simulink library "Arithmetic_Operations_Lib"  (R2023a)
settings: Solver=ode45  StartTime=0.0  StopTime=10.0  RelTol=1e-3  EnableMultiTasking=on
libraries: Miscellaneous x202
(part 1 of 4)
settings Model: Creator=uzivatel  LastModifiedBy=Jozko Mrkvicka
settings SolverCC: AlgebraicLoopSolver=TrustRegion
settings DataIOCC: LimitDataPoints=on  SaveFormat=Array  ReturnWorkspaceOutputs=off
settings OptimizationCC: LifeSpan=inf
settings DebuggingCC: UnderspecifiedInitializationDetection=Classic  MergeDetectMultiDrivingBlocksExec=none  SolverPrmCheckMsg=warning  UnconnectedInputMsg=warning  UnconnectedOutputMsg=warning  UnconnectedLineMsg=warning  StateNameClashWarn=warning  SFUnexpectedBacktrackingDiag=warning  SFNoUnconditionalDefaultTransitionDiag=warning  ArithmeticOperatorsInVariantConditions=warning
settings HardwareCC: ProdBitPerPointer=32  ProdBitPerSizeT=32  ProdBitPerPtrDiffT=32  ProdLargestAtomicFloat=None  ProdIntDivRoundTo=Undefined  ProdEndianess=Unspecified  ProdWordSize=32  ProdHWDeviceType=32-bit Generic
settings ModelReferenceCC: EnableRefExpFcnMdlSchedulingChecks=on  PropagateSignalLabelsOutOfModel=off
settings SFSimCC: SimUseLocalCustomCode=off  CustomCodeUndefinedFunction=UseInterfaceOnly
settings RTWCC: RTWUseLocalCustomCode=off
settings CodeAppCC: StateflowObjectComments=on
settings GRTTargetCC: TargetLangStandard=C89/C90 (ANSI)
settings ConfigComp: CovMetricSettings=dw  CovSaveCumulativeToWorkspaceVar=on  CovSaveSingleToWorkspaceVar=on  CovExternalEMLEnable=off

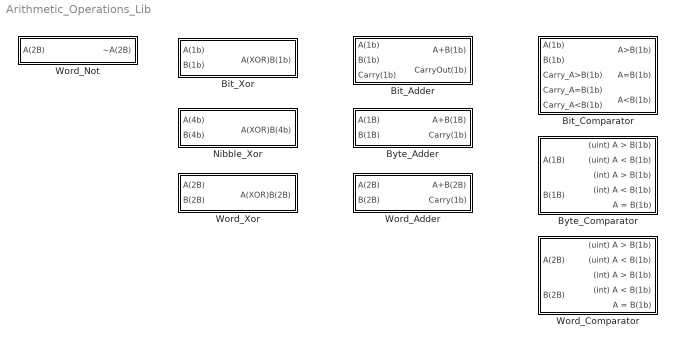
== system Arithmetic_Operations_Lib ==
  Bit_Adder : Subsystem
  Bit_Comparator : Subsystem
  Bit_Xor : Subsystem
  Byte_Adder : Subsystem
  Byte_Comparator : Subsystem
  Nibble_Xor : Subsystem
  Word_Adder : Subsystem
  Word_Comparator : Subsystem
  Word_Not : Subsystem
  Word_Xor : Subsystem

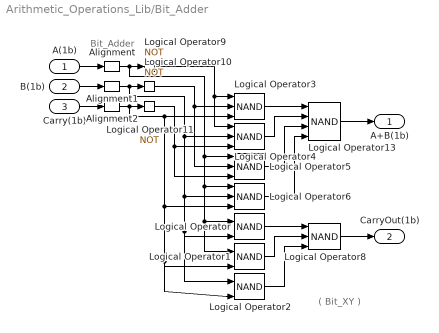
== system Arithmetic_Operations_Lib/Bit_Adder ==
  note: Bit_Adder
  note: ( Bit_XY )
  A(1b) : Inport
  B(1b) : Inport  Port=2
  Carry(1b) : Inport  Port=3
  Alignment : Miscellaneous/Alignment  SystemSampleTime=-1  VariantActivationTime=update diagram  Latency=0  AutoFrameSizeCalculation=off
  Alignment1 : Miscellaneous/Alignment  SystemSampleTime=-1  VariantActivationTime=update diagram  Latency=0  AutoFrameSizeCalculation=off
  Alignment2 : Miscellaneous/Alignment  SystemSampleTime=-1  VariantActivationTime=update diagram  Latency=0  AutoFrameSizeCalculation=off
  Logical Operator : Logic  Operator=NAND  IconShape=distinctive  AllPortsSameDT=off  OutDataTypeStr=boolean
  Logical Operator1 : Logic  Operator=NAND  IconShape=distinctive  AllPortsSameDT=off  OutDataTypeStr=boolean
  Logical Operator10 : Logic  Operator=NOT  Inputs=4  IconShape=distinctive  AllPortsSameDT=off  OutDataTypeStr=boolean
  Logical Operator11 : Logic  Operator=NOT  Inputs=4  IconShape=distinctive  AllPortsSameDT=off  OutDataTypeStr=boolean
  Logical Operator13 : Logic  Operator=NAND  Inputs=4  IconShape=distinctive  AllPortsSameDT=off  OutDataTypeStr=boolean
  Logical Operator2 : Logic  Operator=NAND  IconShape=distinctive  AllPortsSameDT=off  OutDataTypeStr=boolean
  Logical Operator{3..6,8} (5 alike) : Logic  Operator=NAND  Inputs=3  IconShape=distinctive  AllPortsSameDT=off  OutDataTypeStr=boolean
  Logical Operator9 : Logic  Operator=NOT  Inputs=4  IconShape=distinctive  AllPortsSameDT=off  OutDataTypeStr=boolean
  A+B(1b) : Outport
  CarryOut(1b) : Outport  Port=2
  wires:
  Logical Operator11/1 -> Logical Operator5/3, Logical Operator4/3
  Logical Operator10/1 -> Logical Operator5/2, Logical Operator3/2
  Logical Operator9/1 -> Logical Operator4/1, Logical Operator3/1
  A(1b)/1 -> Alignment/1
  B(1b)/1 -> Alignment1/1
  Carry(1b)/1 -> Alignment2/1
  Logical Operator2/1 -> Logical Operator8/3
  Logical Operator1/1 -> Logical Operator8/2
  Logical Operator/1 -> Logical Operator8/1
  Logical Operator8/1 -> CarryOut(1b)/1
  Logical Operator13/1 -> A+B(1b)/1
  Logical Operator6/1 -> Logical Operator13/4
  Logical Operator5/1 -> Logical Operator13/3
  Logical Operator4/1 -> Logical Operator13/2
  Logical Operator3/1 -> Logical Operator13/1
  Alignment/1 -> Logical Operator1/1, Logical Operator/1, Logical Operator6/1, Logical Operator5/1, Logical Operator9/1
  Alignment1/1 -> Logical Operator10/1, Logical Operator2/1, Logical Operator/2, Logical Operator6/2, Logical Operator4/2
  Alignment2/1 -> Logical Operator11/1, Logical Operator2/2, Logical Operator1/2, Logical Operator6/3, Logical Operator3/3

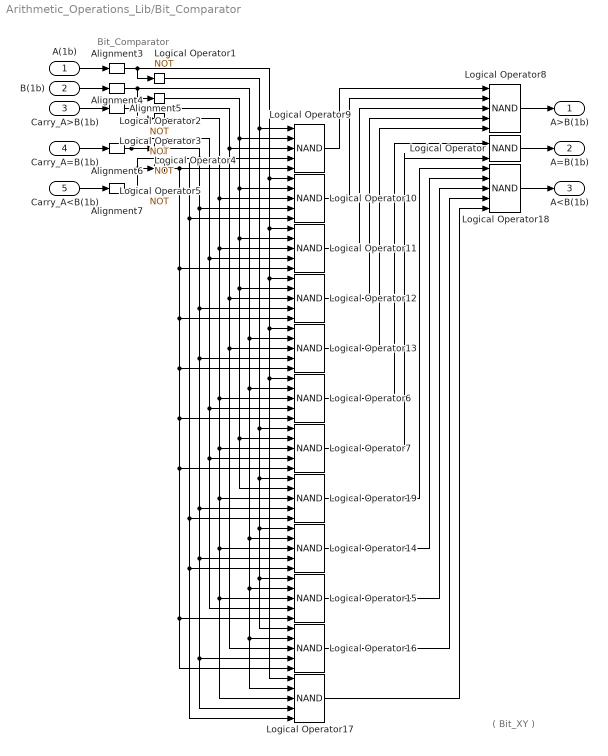
== system Arithmetic_Operations_Lib/Bit_Comparator ==
  note: Bit_Comparator
  note: ( Bit_XY )
  A(1b) : Inport
  B(1b) : Inport  Port=2
  Carry_A>B(1b) : Inport  Port=3
  Carry_A=B(1b) : Inport  Port=4
  Carry_A<B(1b) : Inport  Port=5
  Alignment{3..7} (5 alike) : Miscellaneous/Alignment  SystemSampleTime=-1  VariantActivationTime=update diagram  Latency=0  AutoFrameSizeCalculation=off
  Logical Operator : Logic  Operator=NAND  IconShape=distinctive  AllPortsSameDT=off  OutDataTypeStr=boolean
  Logical Operator{1..5} (5 alike) : Logic  Operator=NOT  IconShape=distinctive  AllPortsSameDT=off  OutDataTypeStr=boolean
  Logical Operator{6..19} (14 alike) : Logic  Operator=NAND  Inputs=5  IconShape=distinctive  AllPortsSameDT=off  OutDataTypeStr=boolean
  A>B(1b) : Outport
  A=B(1b) : Outport  Port=2
  A<B(1b) : Outport  Port=3
  wires:
  Logical Operator16/1 -> Logical Operator18/4
  Logical Operator17/1 -> Logical Operator18/5
  Logical Operator19/1 -> Logical Operator18/1
  Logical Operator15/1 -> Logical Operator18/3
  Logical Operator14/1 -> Logical Operator18/2
  Logical Operator4/1 -> Logical Operator10/4, Logical Operator12/4, Logical Operator13/4, Logical Operator19/4, Logical Operator14/4, Logical Operator17/4, Logical Operator16/4, Logical Operator9/4
  A(1b)/1 -> Alignment3/1
  Logical Operator5/1 -> Logical Operator11/5, Logical Operator12/5, Logical Operator13/5, Logical Operator6/5, Logical Operator7/5, Logical Operator16/5, Logical Operator15/5, Logical Operator9/5
  Logical Operator2/1 -> Logical Operator10/2, Logical Operator11/2, Logical Operator12/2, Logical Operator19/2, Logical Operator7/2, Logical Operator9/2
  Logical Operator1/1 -> Logical Operator7/1, Logical Operator19/1, Logical Operator14/1, Logical Operator15/1, Logical Operator16/1, Logical Operator9/1
  Logical Operator3/1 -> Logical Operator10/3, Logical Operator11/3, Logical Operator6/3, Logical Operator7/3, Logical Operator19/3, Logical Operator14/3, Logical Operator17/3, Logical Operator15/3
  Carry_A<B(1b)/1 -> Alignment7/1
  Carry_A>B(1b)/1 -> Alignment5/1
  Carry_A=B(1b)/1 -> Alignment6/1
  Logical Operator6/1 -> Logical Operator/1
  Logical Operator7/1 -> Logical Operator/2
  B(1b)/1 -> Alignment4/1
  Logical Operator13/1 -> Logical Operator8/5
  Logical Operator11/1 -> Logical Operator8/3
  Logical Operator10/1 -> Logical Operator8/2
  Logical Operator12/1 -> Logical Operator8/4
  Logical Operator9/1 -> Logical Operator8/1
  Alignment3/1 -> Logical Operator10/1, Logical Operator11/1, Logical Operator12/1, Logical Operator13/1, Logical Operator6/1, Logical Operator17/1, Logical Operator1/1
  Alignment4/1 -> Logical Operator2/1, Logical Operator13/2, Logical Operator6/2, Logical Operator14/2, Logical Operator15/2, Logical Operator17/2, Logical Operator16/2
  Alignment5/1 -> Logical Operator3/1, Logical Operator12/3, Logical Operator16/3, Logical Operator13/3, Logical Operator9/3
  Alignment6/1 -> Logical Operator4/1, Logical Operator11/4, Logical Operator6/4, Logical Operator7/4, Logical Operator15/4
  Alignment7/1 -> Logical Operator10/5, Logical Operator19/5, Logical Operator17/5, Logical Operator14/5, Logical Operator5/1
  Logical Operator/1 -> A=B(1b)/1
  Logical Operator8/1 -> A>B(1b)/1
  Logical Operator18/1 -> A<B(1b)/1

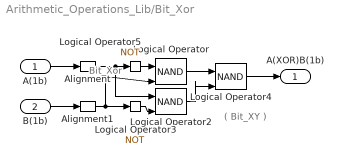
== system Arithmetic_Operations_Lib/Bit_Xor ==
  note: Bit_Xor
  note: ( Bit_XY )
  A(1b) : Inport
  B(1b) : Inport  Port=2
  Alignment : Miscellaneous/Alignment  SystemSampleTime=-1  VariantActivationTime=update diagram  Latency=0  AutoFrameSizeCalculation=off
  Alignment1 : Miscellaneous/Alignment  SystemSampleTime=-1  VariantActivationTime=update diagram  Latency=0  AutoFrameSizeCalculation=off
  Logical Operator : Logic  Operator=NAND  IconShape=distinctive  AllPortsSameDT=off  OutDataTypeStr=boolean
  Logical Operator2 : Logic  Operator=NAND  IconShape=distinctive  AllPortsSameDT=off  OutDataTypeStr=boolean
  Logical Operator3 : Logic  Operator=NOT  IconShape=distinctive  AllPortsSameDT=off  OutDataTypeStr=boolean
  Logical Operator4 : Logic  Operator=NAND  IconShape=distinctive  AllPortsSameDT=off  OutDataTypeStr=boolean
  Logical Operator5 : Logic  Operator=NOT  IconShape=distinctive  AllPortsSameDT=off  OutDataTypeStr=boolean
  A(XOR)B(1b) : Outport
  wires:
  Logical Operator3/1 -> Logical Operator2/2
  A(1b)/1 -> Alignment/1
  B(1b)/1 -> Alignment1/1
  Logical Operator4/1 -> A(XOR)B(1b)/1
  Logical Operator2/1 -> Logical Operator4/2
  Logical Operator5/1 -> Logical Operator/1
  Logical Operator/1 -> Logical Operator4/1
  Alignment/1 -> Logical Operator2/1, Logical Operator5/1
  Alignment1/1 -> Logical Operator3/1, Logical Operator/2

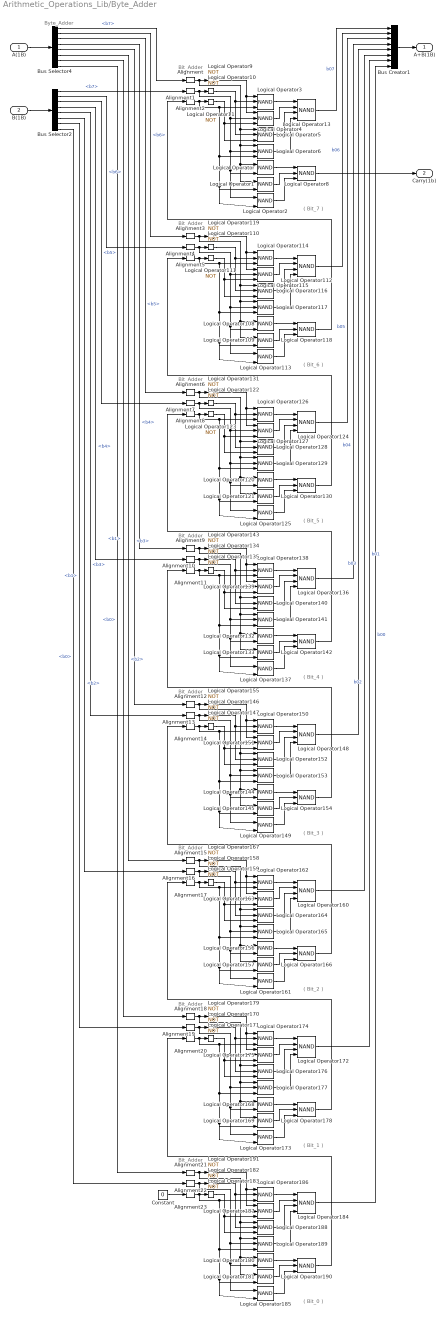
== system Arithmetic_Operations_Lib/Byte_Adder ==
  note: Byte_Adder
  note: Bit_Adder
  note: ( Bit_7 )
  note: Bit_Adder
  note: ( Bit_6 )
  note: Bit_Adder
  note: ( Bit_5 )
  note: Bit_Adder
  note: ( Bit_4 )
  note: Bit_Adder
  note: ( Bit_3 )
  note: Bit_Adder
  note: ( Bit_2 )
  note: Bit_Adder
  note: ( Bit_1 )
  note: Bit_Adder
  note: ( Bit_0 )
  A(1B) : Inport
  B(1B) : Inport  Port=2
  Alignment{,1..23} (24 alike) : Miscellaneous/Alignment  SystemSampleTime=-1  VariantActivationTime=update diagram  Latency=0  AutoFrameSizeCalculation=off
  Bus Creator1 : BusCreator  Inputs=8
  Bus Selector2 : BusSelector  OutputSignals=b7,b6,b5,b4,b3,b2,b1,b0
  Bus Selector4 : BusSelector  OutputSignals=b7,b6,b5,b4,b3,b2,b1,b0
  Constant : Constant  Value=0
  Logical Operator{,1..2,108..109,113,120..121,125,132..133,137,144..145,149,156..157,161,168..169,173,180..181,185} (24 alike) : Logic  Operator=NAND  IconShape=distinctive  AllPortsSameDT=off  OutDataTypeStr=boolean
  Logical Operator{9..11,110..111,119,122..123,131,134..135,143,146..147,155,158..159,167,170..171,179,182..183,191} (24 alike) : Logic  Operator=NOT  Inputs=4  IconShape=distinctive  AllPortsSameDT=off  OutDataTypeStr=boolean
  Logical Operator{13,112,124,136,148,160,172,184} (8 alike) : Logic  Operator=NAND  Inputs=4  IconShape=distinctive  AllPortsSameDT=off  OutDataTypeStr=boolean
  Logical Operator{3..6,8,114..118,126..130,138..142,150..154,162..166,174..178,186..190} (40 alike) : Logic  Operator=NAND  Inputs=3  IconShape=distinctive  AllPortsSameDT=off  OutDataTypeStr=boolean
  A+B(1B) : Outport
  Carry(1b) : Outport  Port=2
  wires:
  Bus Selector4/3 -> Alignment6/1  "<b5>"
  Bus Selector2/6 -> Alignment16/1  "<b2>"
  Bus Selector2/8 -> Alignment22/1  "<b0>"
  Bus Selector2/5 -> Alignment13/1  "<b3>"
  Bus Selector4/8 -> Alignment21/1  "<b0>"
  Bus Selector4/4 -> Alignment9/1  "<b4>"
  Bus Selector2/1 -> Alignment1/1  "<b7>"
  Bus Selector2/3 -> Alignment7/1  "<b5>"
  Bus Selector4/7 -> Alignment18/1  "<b1>"
  Bus Selector2/2 -> Alignment4/1  "<b6>"
  Logical Operator172/1 -> Bus Creator1/7  "b01"
  Logical Operator13/1 -> Bus Creator1/1  "b07"
  Bus Selector4/6 -> Alignment15/1  "<b2>"
  Logical Operator184/1 -> Bus Creator1/8  "b00"
  Logical Operator124/1 -> Bus Creator1/3  "b05"
  Bus Selector2/7 -> Alignment19/1  "<b1>"
  Logical Operator112/1 -> Bus Creator1/2  "b06"
  Logical Operator148/1 -> Bus Creator1/5  "b03"
  Bus Selector4/2 -> Alignment3/1  "<b6>"
  Logical Operator136/1 -> Bus Creator1/4  "b04"
  Bus Selector4/5 -> Alignment12/1  "<b3>"
  Logical Operator8/1 -> Carry(1b)/1
  Logical Operator160/1 -> Bus Creator1/6  "b02"
  Bus Selector4/1 -> Alignment/1  "<b7>"
  Bus Selector2/4 -> Alignment10/1  "<b4>"
  Logical Operator11/1 -> Logical Operator4/3, Logical Operator5/3
  Logical Operator10/1 -> Logical Operator3/2, Logical Operator5/2
  Logical Operator9/1 -> Logical Operator4/1, Logical Operator3/1
  Logical Operator118/1 -> Alignment2/1
  Logical Operator2/1 -> Logical Operator8/3
  Logical Operator1/1 -> Logical Operator8/2
  Logical Operator/1 -> Logical Operator8/1
  Logical Operator6/1 -> Logical Operator13/4
  Logical Operator5/1 -> Logical Operator13/3
  Logical Operator4/1 -> Logical Operator13/2
  Logical Operator3/1 -> Logical Operator13/1
  Alignment/1 -> Logical Operator9/1, Logical Operator5/1, Logical Operator6/1, Logical Operator/1, Logical Operator1/1
  Alignment1/1 -> Logical Operator4/2, Logical Operator6/2, Logical Operator/2, Logical Operator2/1, Logical Operator10/1
  Alignment2/1 -> Logical Operator3/3, Logical Operator6/3, Logical Operator1/2, Logical Operator2/2, Logical Operator11/1
  Logical Operator111/1 -> Logical Operator115/3, Logical Operator116/3
  Logical Operator110/1 -> Logical Operator114/2, Logical Operator116/2
  Logical Operator119/1 -> Logical Operator115/1, Logical Operator114/1
  Logical Operator130/1 -> Alignment5/1
  Logical Operator113/1 -> Logical Operator118/3
  Logical Operator109/1 -> Logical Operator118/2
  Logical Operator108/1 -> Logical Operator118/1
  Logical Operator117/1 -> Logical Operator112/4
  Logical Operator116/1 -> Logical Operator112/3
  Logical Operator115/1 -> Logical Operator112/2
  Logical Operator114/1 -> Logical Operator112/1
  Alignment3/1 -> Logical Operator119/1, Logical Operator109/1, Logical Operator108/1, Logical Operator117/1, Logical Operator116/1
  Alignment4/1 -> Logical Operator115/2, Logical Operator117/2, Logical Operator108/2, Logical Operator113/1, Logical Operator110/1
  Alignment5/1 -> Logical Operator114/3, Logical Operator117/3, Logical Operator109/2, Logical Operator113/2, Logical Operator111/1
  Logical Operator123/1 -> Logical Operator127/3, Logical Operator128/3
  Logical Operator122/1 -> Logical Operator126/2, Logical Operator128/2
  Logical Operator131/1 -> Logical Operator127/1, Logical Operator126/1
  Logical Operator142/1 -> Alignment8/1
  Logical Operator125/1 -> Logical Operator130/3
  Logical Operator121/1 -> Logical Operator130/2
  Logical Operator120/1 -> Logical Operator130/1
  Logical Operator129/1 -> Logical Operator124/4
  Logical Operator128/1 -> Logical Operator124/3
  Logical Operator127/1 -> Logical Operator124/2
  Logical Operator126/1 -> Logical Operator124/1
  Alignment6/1 -> Logical Operator131/1, Logical Operator121/1, Logical Operator120/1, Logical Operator129/1, Logical Operator128/1
  Alignment7/1 -> Logical Operator125/1, Logical Operator120/2, Logical Operator129/2, Logical Operator127/2, Logical Operator122/1
  Alignment8/1 -> Logical Operator126/3, Logical Operator129/3, Logical Operator121/2, Logical Operator125/2, Logical Operator123/1
  Logical Operator135/1 -> Logical Operator139/3, Logical Operator140/3
  Logical Operator134/1 -> Logical Operator138/2, Logical Operator140/2
  Logical Operator143/1 -> Logical Operator139/1, Logical Operator138/1
  Logical Operator154/1 -> Alignment11/1
  Logical Operator137/1 -> Logical Operator142/3
  Logical Operator133/1 -> Logical Operator142/2
  Logical Operator132/1 -> Logical Operator142/1
  Logical Operator141/1 -> Logical Operator136/4
  Logical Operator140/1 -> Logical Operator136/3
  Logical Operator139/1 -> Logical Operator136/2
  Logical Operator138/1 -> Logical Operator136/1
  Alignment9/1 -> Logical Operator143/1, Logical Operator140/1, Logical Operator141/1, Logical Operator132/1, Logical Operator133/1
  Alignment10/1 -> Logical Operator139/2, Logical Operator141/2, Logical Operator132/2, Logical Operator137/1, Logical Operator134/1
  Alignment11/1 -> Logical Operator138/3, Logical Operator141/3, Logical Operator133/2, Logical Operator137/2, Logical Operator135/1
  Logical Operator147/1 -> Logical Operator151/3, Logical Operator152/3
  Logical Operator146/1 -> Logical Operator150/2, Logical Operator152/2
  Logical Operator155/1 -> Logical Operator151/1, Logical Operator150/1
  Logical Operator166/1 -> Alignment14/1
  Logical Operator149/1 -> Logical Operator154/3
  Logical Operator145/1 -> Logical Operator154/2
  Logical Operator144/1 -> Logical Operator154/1
  Logical Operator153/1 -> Logical Operator148/4
  Logical Operator152/1 -> Logical Operator148/3
  Logical Operator151/1 -> Logical Operator148/2
  Logical Operator150/1 -> Logical Operator148/1
  Alignment12/1 -> Logical Operator155/1, Logical Operator152/1, Logical Operator153/1, Logical Operator144/1, Logical Operator145/1
  Alignment13/1 -> Logical Operator151/2, Logical Operator153/2, Logical Operator144/2, Logical Operator149/1, Logical Operator146/1
  Alignment14/1 -> Logical Operator150/3, Logical Operator153/3, Logical Operator145/2, Logical Operator149/2, Logical Operator147/1
  Logical Operator159/1 -> Logical Operator163/3, Logical Operator164/3
  Logical Operator158/1 -> Logical Operator162/2, Logical Operator164/2
  Logical Operator167/1 -> Logical Operator163/1, Logical Operator162/1
  Logical Operator178/1 -> Alignment17/1
  Logical Operator161/1 -> Logical Operator166/3
  Logical Operator157/1 -> Logical Operator166/2
  Logical Operator156/1 -> Logical Operator166/1
  Logical Operator165/1 -> Logical Operator160/4
  Logical Operator164/1 -> Logical Operator160/3
  Logical Operator163/1 -> Logical Operator160/2
  Logical Operator162/1 -> Logical Operator160/1
  Alignment15/1 -> Logical Operator167/1, Logical Operator164/1, Logical Operator165/1, Logical Operator156/1, Logical Operator157/1
  Alignment16/1 -> Logical Operator163/2, Logical Operator165/2, Logical Operator156/2, Logical Operator161/1, Logical Operator158/1
  Alignment17/1 -> Logical Operator162/3, Logical Operator165/3, Logical Operator157/2, Logical Operator161/2, Logical Operator159/1
  Logical Operator171/1 -> Logical Operator175/3, Logical Operator176/3
  Logical Operator170/1 -> Logical Operator174/2, Logical Operator176/2
  Logical Operator179/1 -> Logical Operator175/1, Logical Operator174/1
  Logical Operator190/1 -> Alignment20/1
  Logical Operator173/1 -> Logical Operator178/3
  Logical Operator169/1 -> Logical Operator178/2
  Logical Operator168/1 -> Logical Operator178/1
  Logical Operator177/1 -> Logical Operator172/4
  Logical Operator176/1 -> Logical Operator172/3
  Logical Operator175/1 -> Logical Operator172/2
  Logical Operator174/1 -> Logical Operator172/1
  Alignment18/1 -> Logical Operator179/1, Logical Operator176/1, Logical Operator177/1, Logical Operator168/1, Logical Operator169/1
  Alignment19/1 -> Logical Operator175/2, Logical Operator177/2, Logical Operator168/2, Logical Operator173/1, Logical Operator170/1
  Alignment20/1 -> Logical Operator174/3, Logical Operator177/3, Logical Operator169/2, Logical Operator173/2, Logical Operator171/1
  Logical Operator183/1 -> Logical Operator187/3, Logical Operator188/3
  Logical Operator182/1 -> Logical Operator186/2, Logical Operator188/2
  Logical Operator191/1 -> Logical Operator187/1, Logical Operator186/1
  Constant/1 -> Alignment23/1
  Logical Operator185/1 -> Logical Operator190/3
  Logical Operator181/1 -> Logical Operator190/2
  Logical Operator180/1 -> Logical Operator190/1
  Logical Operator189/1 -> Logical Operator184/4
  Logical Operator188/1 -> Logical Operator184/3
  Logical Operator187/1 -> Logical Operator184/2
  Logical Operator186/1 -> Logical Operator184/1
  Alignment21/1 -> Logical Operator191/1, Logical Operator188/1, Logical Operator189/1, Logical Operator180/1, Logical Operator181/1
  Alignment22/1 -> Logical Operator187/2, Logical Operator189/2, Logical Operator180/2, Logical Operator185/1, Logical Operator182/1
  Alignment23/1 -> Logical Operator186/3, Logical Operator189/3, Logical Operator181/2, Logical Operator185/2, Logical Operator183/1
  B(1B)/1 -> Bus Selector2/1
  A(1B)/1 -> Bus Selector4/1
  Bus Creator1/1 -> A+B(1B)/1

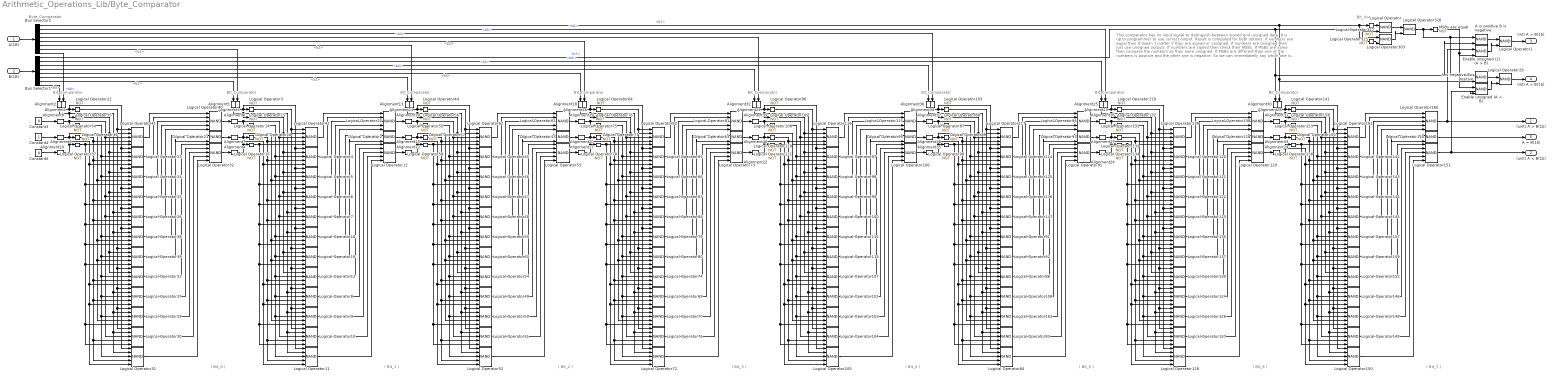
== system Arithmetic_Operations_Lib/Byte_Comparator ==
  note: Byte_Comparator
  note: This comparator has no input signal to distinguish between signed and unsigned data. It is up to programmer to use correct output. Result is computed for both options.
      | If numbers are equal then it doesn`t matter if they are signed or unsigned.
      | If numbers are unsigned then just use unsigned outputs.
      | If numbers are signed then check their MSBs.
      | If MSBs are same then compare the numbers as they were unsigned.
      | If MSBs are different then one of the numbers is positive and the other one is negative. So we can immediatelly say which one is greater.
  note: Bit_Comparator
  note: ( Bit_0 )
  note: ( Bit_1 )
  note: Bit_Comparator
  note: ( Bit_2 )
  note: Bit_Comparator
  note: ( Bit_3 )
  note: Bit_Comparator
  note: ( Bit_6 )
  note: Bit_Comparator
  note: ( Bit_5 )
  note: ( Bit_4 )
  note: Bit_Comparator
  note: Bit_Comparator
  note: Bit_Comparator
  note: ( Bit_7 )
  note: Bit_Xor
  A(1B) : Inport
  B(1B) : Inport  Port=2
  "A is negative B is positive " : Logic  Operator=NAND  IconShape=distinctive  AllPortsSameDT=off  OutDataTypeStr=boolean
  A is positive B is negative : Logic  Operator=NAND  IconShape=distinctive  AllPortsSameDT=off  OutDataTypeStr=boolean
  Alignment{1..40} (40 alike) : Miscellaneous/Alignment  SystemSampleTime=-1  VariantActivationTime=update diagram  Latency=0  AutoFrameSizeCalculation=off
  Bus Selector1 : BusSelector  OutputSignals=b7,b6,b5,b4,b3,b2,b1,b0
  Bus Selector2 : BusSelector  OutputSignals=b7,b6,b5,b4,b3,b2,b1,b0
  Constant3 : Constant  Value=0  OutDataTypeStr=int16
  Constant4 : Constant  OutDataTypeStr=int16
  Constant5 : Constant  Value=0  OutDataTypeStr=int16
  Enable unsigned (A < B) : Logic  Operator=NAND  IconShape=distinctive  AllPortsSameDT=off  OutDataTypeStr=boolean
  Enable unsigned (2) (A > B) : Logic  Operator=NAND  IconShape=distinctive  AllPortsSameDT=off  OutDataTypeStr=boolean
  Logical Operator{,1..2,21,29,43,63,93,95,118,140,303,326} (13 alike) : Logic  Operator=NAND  IconShape=distinctive  AllPortsSameDT=off  OutDataTypeStr=boolean
  Logical Operator{4..13,18..20,23..28,30..33,38..42,45..54,59..62,65..74,79..86,91..92,94,97..102,104..107,112..117,120..130,135..139,142..152,157..162} (112 alike) : Logic  Operator=NAND  Inputs=5  IconShape=distinctive  AllPortsSameDT=off  OutDataTypeStr=boolean
  Logical Operator{3,14..17,22,34..37,44,55..58,64,75..78,87..90,96,103,108..111,119,131..134,141,153..156,325,327} (42 alike) : Logic  Operator=NOT  IconShape=distinctive  AllPortsSameDT=off  OutDataTypeStr=boolean
  MSBs are equal : Logic  Operator=NOT  IconShape=distinctive  AllPortsSameDT=off  OutDataTypeStr=boolean
  (uint) A > B(1b) : Outport
  (uint) A < B(1b) : Outport  Port=2
  (int) A > B(1b) : Outport  Port=3
  (int) A < B(1b) : Outport  Port=4
  A = B(1b) : Outport  Port=5
  wires:
  Bus Selector2/7 -> Alignment3/1  "<b1>"
  Bus Selector1/7 -> Alignment5/1  "<b1>"
  "A is negative B is positive "/1 -> Logical Operator29/1
  A is positive B is negative/1 -> Logical Operator1/1
  Logical Operator29/1 -> (int) A < B(1b)/1
  Logical Operator1/1 -> (int) A > B(1b)/1
  Enable unsigned (A < B)/1 -> Logical Operator29/2
  Enable unsigned (2) (A > B)/1 -> Logical Operator1/2
  MSBs are equal/1 -> Enable unsigned (A < B)/1, Enable unsigned (2) (A > B)/2
  Logical Operator326/1 -> MSBs are equal/1, A is positive B is negative/1, "A is negative B is positive "/1
  Constant5/1 -> Alignment10/1
  Constant3/1 -> Alignment8/1
  Constant4/1 -> Alignment9/1
  Logical Operator30/1 -> Logical Operator32/4
  Logical Operator31/1 -> Logical Operator32/5
  Logical Operator33/1 -> Logical Operator32/1
  Logical Operator28/1 -> Logical Operator32/3
  Logical Operator27/1 -> Logical Operator32/2
  Logical Operator36/1 -> Logical Operator41/4, Logical Operator30/4, Logical Operator31/4, Logical Operator27/4, Logical Operator33/4, Logical Operator26/4, Logical Operator25/4, Logical Operator23/4
  Logical Operator37/1 -> Logical Operator41/5, Logical Operator28/5, Logical Operator30/5, Logical Operator39/5, Logical Operator38/5, Logical Operator26/5, Logical Operator25/5, Logical Operator24/5
  Logical Operator34/1 -> Logical Operator41/2, Logical Operator39/2, Logical Operator33/2, Logical Operator25/2, Logical Operator24/2, Logical Operator23/2
  Logical Operator22/1 -> Logical Operator41/1, Logical Operator30/1, Logical Operator28/1, Logical Operator27/1, Logical Operator33/1, Logical Operator39/1
  Logical Operator35/1 -> Logical Operator28/3, Logical Operator31/3, Logical Operator27/3, Logical Operator33/3, Logical Operator39/3, Logical Operator38/3, Logical Operator24/3, Logical Operator23/3
  Logical Operator38/1 -> Logical Operator21/1
  Logical Operator39/1 -> Logical Operator21/2
  Logical Operator26/1 -> Logical Operator40/5
  Logical Operator24/1 -> Logical Operator40/3
  Logical Operator23/1 -> Logical Operator40/2
  Logical Operator25/1 -> Logical Operator40/4
  Logical Operator41/1 -> Logical Operator40/1
  Alignment1/1 -> Logical Operator31/1, Logical Operator38/1, Logical Operator26/1, Logical Operator25/1, Logical Operator24/1, Logical Operator23/1, Logical Operator22/1
  Alignment2/1 -> Logical Operator30/2, Logical Operator31/2, Logical Operator28/2, Logical Operator27/2, Logical Operator38/2, Logical Operator26/2, Logical Operator34/1
  Alignment8/1 -> Logical Operator41/3, Logical Operator26/3, Logical Operator30/3, Logical Operator25/3, Logical Operator35/1
  Alignment9/1 -> Logical Operator36/1, Logical Operator28/4, Logical Operator39/4, Logical Operator38/4, Logical Operator24/4
  Alignment10/1 -> Logical Operator37/1, Logical Operator27/5, Logical Operator31/5, Logical Operator33/5, Logical Operator23/5
  Logical Operator42/1 -> Logical Operator20/1
  Logical Operator6/1 -> Logical Operator20/4
  Alignment3/1 -> Logical Operator11/1, Logical Operator18/1, Logical Operator7/1, Logical Operator6/1, Logical Operator5/1, Logical Operator4/1, Logical Operator3/1
  Logical Operator14/1 -> Logical Operator42/2, Logical Operator19/2, Logical Operator13/2, Logical Operator6/2, Logical Operator5/2, Logical Operator4/2
  Logical Operator3/1 -> Logical Operator42/1, Logical Operator10/1, Logical Operator9/1, Logical Operator8/1, Logical Operator13/1, Logical Operator19/1
  Logical Operator17/1 -> Logical Operator42/5, Logical Operator9/5, Logical Operator10/5, Logical Operator19/5, Logical Operator18/5, Logical Operator7/5, Logical Operator6/5, Logical Operator5/5
  Logical Operator15/1 -> Logical Operator9/3, Logical Operator11/3, Logical Operator8/3, Logical Operator13/3, Logical Operator19/3, Logical Operator18/3, Logical Operator5/3, Logical Operator4/3
  Logical Operator16/1 -> Logical Operator42/4, Logical Operator10/4, Logical Operator11/4, Logical Operator8/4, Logical Operator13/4, Logical Operator7/4, Logical Operator6/4, Logical Operator4/4
  Logical Operator9/1 -> Logical Operator12/3
  Logical Operator10/1 -> Logical Operator12/4
  Logical Operator18/1 -> Logical Operator2/1
  Logical Operator7/1 -> Logical Operator20/5
  Logical Operator13/1 -> Logical Operator12/1
  Alignment7/1 -> Logical Operator16/1, Logical Operator9/4, Logical Operator19/4, Logical Operator18/4, Logical Operator5/4
  Logical Operator11/1 -> Logical Operator12/5
  Alignment4/1 -> Logical Operator17/1, Logical Operator8/5, Logical Operator11/5, Logical Operator13/5, Logical Operator4/5
  Alignment5/1 -> Logical Operator10/2, Logical Operator11/2, Logical Operator9/2, Logical Operator8/2, Logical Operator18/2, Logical Operator7/2, Logical Operator14/1
  Logical Operator19/1 -> Logical Operator2/2
  Alignment6/1 -> Logical Operator42/3, Logical Operator7/3, Logical Operator10/3, Logical Operator6/3, Logical Operator15/1
  Logical Operator8/1 -> Logical Operator12/2
  Logical Operator5/1 -> Logical Operator20/3
  Logical Operator4/1 -> Logical Operator20/2
  Logical Operator62/1 -> Logical Operator61/1
  Logical Operator47/1 -> Logical Operator61/4
  Alignment11/1 -> Logical Operator52/1, Logical Operator59/1, Logical Operator48/1, Logical Operator47/1, Logical Operator46/1, Logical Operator45/1, Logical Operator44/1
  Logical Operator55/1 -> Logical Operator62/2, Logical Operator60/2, Logical Operator54/2, Logical Operator47/2, Logical Operator46/2, Logical Operator45/2
  Logical Operator44/1 -> Logical Operator62/1, Logical Operator51/1, Logical Operator50/1, Logical Operator49/1, Logical Operator54/1, Logical Operator60/1
  Logical Operator58/1 -> Logical Operator62/5, Logical Operator50/5, Logical Operator51/5, Logical Operator60/5, Logical Operator59/5, Logical Operator48/5, Logical Operator47/5, Logical Operator46/5
  Logical Operator56/1 -> Logical Operator50/3, Logical Operator52/3, Logical Operator49/3, Logical Operator54/3, Logical Operator60/3, Logical Operator59/3, Logical Operator46/3, Logical Operator45/3
  Logical Operator57/1 -> Logical Operator62/4, Logical Operator51/4, Logical Operator52/4, Logical Operator49/4, Logical Operator54/4, Logical Operator48/4, Logical Operator47/4, Logical Operator45/4
  Logical Operator50/1 -> Logical Operator53/3
  Logical Operator51/1 -> Logical Operator53/4
  Logical Operator59/1 -> Logical Operator43/1
  Logical Operator48/1 -> Logical Operator61/5
  Logical Operator54/1 -> Logical Operator53/1
  Alignment15/1 -> Logical Operator57/1, Logical Operator50/4, Logical Operator60/4, Logical Operator59/4, Logical Operator46/4
  Logical Operator52/1 -> Logical Operator53/5
  Alignment12/1 -> Logical Operator58/1, Logical Operator49/5, Logical Operator52/5, Logical Operator54/5, Logical Operator45/5
  Alignment13/1 -> Logical Operator51/2, Logical Operator52/2, Logical Operator50/2, Logical Operator49/2, Logical Operator59/2, Logical Operator48/2, Logical Operator55/1
  Logical Operator60/1 -> Logical Operator43/2
  Alignment14/1 -> Logical Operator62/3, Logical Operator48/3, Logical Operator51/3, Logical Operator47/3, Logical Operator56/1
  Logical Operator49/1 -> Logical Operator53/2
  Logical Operator46/1 -> Logical Operator61/3
  Logical Operator45/1 -> Logical Operator61/2
  Logical Operator82/1 -> Logical Operator81/1
  Logical Operator67/1 -> Logical Operator81/4
  Alignment16/1 -> Logical Operator72/1, Logical Operator79/1, Logical Operator68/1, Logical Operator67/1, Logical Operator66/1, Logical Operator65/1, Logical Operator64/1
  Logical Operator75/1 -> Logical Operator82/2, Logical Operator80/2, Logical Operator74/2, Logical Operator67/2, Logical Operator66/2, Logical Operator65/2
  Logical Operator64/1 -> Logical Operator82/1, Logical Operator71/1, Logical Operator70/1, Logical Operator69/1, Logical Operator74/1, Logical Operator80/1
  Logical Operator78/1 -> Logical Operator82/5, Logical Operator70/5, Logical Operator71/5, Logical Operator80/5, Logical Operator79/5, Logical Operator68/5, Logical Operator67/5, Logical Operator66/5
  Logical Operator76/1 -> Logical Operator70/3, Logical Operator72/3, Logical Operator69/3, Logical Operator74/3, Logical Operator80/3, Logical Operator79/3, Logical Operator66/3, Logical Operator65/3
  Logical Operator77/1 -> Logical Operator82/4, Logical Operator71/4, Logical Operator72/4, Logical Operator69/4, Logical Operator74/4, Logical Operator68/4, Logical Operator67/4, Logical Operator65/4
  Logical Operator70/1 -> Logical Operator73/3
  Logical Operator71/1 -> Logical Operator73/4
  Logical Operator79/1 -> Logical Operator63/1
  Logical Operator68/1 -> Logical Operator81/5
  Logical Operator74/1 -> Logical Operator73/1
  Alignment20/1 -> Logical Operator77/1, Logical Operator70/4, Logical Operator80/4, Logical Operator79/4, Logical Operator66/4
  Logical Operator72/1 -> Logical Operator73/5
  Alignment17/1 -> Logical Operator78/1, Logical Operator69/5, Logical Operator72/5, Logical Operator74/5, Logical Operator65/5
  Alignment18/1 -> Logical Operator71/2, Logical Operator72/2, Logical Operator70/2, Logical Operator69/2, Logical Operator79/2, Logical Operator68/2, Logical Operator75/1
  Logical Operator80/1 -> Logical Operator63/2
  Alignment19/1 -> Logical Operator82/3, Logical Operator68/3, Logical Operator71/3, Logical Operator67/3, Logical Operator76/1
  Logical Operator69/1 -> Logical Operator73/2
  Logical Operator66/1 -> Logical Operator81/3
  Logical Operator65/1 -> Logical Operator81/2
  Logical Operator61/1 -> Alignment19/1
  Logical Operator43/1 -> Alignment20/1
  Logical Operator53/1 -> Alignment17/1
  Logical Operator20/1 -> Alignment14/1
  Logical Operator2/1 -> Alignment15/1
  Logical Operator12/1 -> Alignment12/1
  Logical Operator40/1 -> Alignment6/1
  Logical Operator21/1 -> Alignment7/1
  Logical Operator32/1 -> Alignment4/1
  Logical Operator145/1 -> Logical Operator160/5
  Logical Operator157/1 -> Logical Operator140/1
  Logical Operator152/1 -> Logical Operator151/1
  Logical Operator149/1 -> Logical Operator151/4
  Logical Operator154/1 -> Logical Operator148/3, Logical Operator150/3, Logical Operator146/3, Logical Operator152/3, Logical Operator159/3, Logical Operator157/3, Logical Operator143/3, Logical Operator142/3
  Logical Operator155/1 -> Logical Operator161/4, Logical Operator149/4, Logical Operator150/4, Logical Operator146/4, Logical Operator152/4, Logical Operator145/4, Logical Operator144/4, Logical Operator142/4
  Logical Operator148/1 -> Logical Operator151/3
  Alignment28/1 -> Logical Operator150/1, Logical Operator157/1, Logical Operator145/1, Logical Operator144/1, Logical Operator143/1, Logical Operator142/1, Logical Operator141/1
  Logical Operator144/1 -> Logical Operator160/4
  Logical Operator118/1 -> Alignment33/1
  Logical Operator106/1 -> Alignment35/1
  Logical Operator117/1 -> Logical Operator94/1
  Logical Operator161/1 -> Logical Operator160/1
  Logical Operator129/1 -> Alignment29/1
  Logical Operator124/1 -> Logical Operator129/2
  Alignment26/1 -> Logical Operator139/3, Logical Operator123/3, Logical Operator127/3, Logical Operator122/3, Logical Operator132/1
  Alignment25/1 -> Logical Operator127/2, Logical Operator128/2, Logical Operator126/2, Logical Operator124/2, Logical Operator135/2, Logical Operator123/2, Logical Operator131/1
  Logical Operator137/1 -> Logical Operator118/2
  Alignment27/1 -> Logical Operator133/1, Logical Operator126/4, Logical Operator137/4, Logical Operator135/4, Logical Operator121/4
  Alignment24/1 -> Logical Operator134/1, Logical Operator124/5, Logical Operator128/5, Logical Operator130/5, Logical Operator120/5
  Logical Operator128/1 -> Logical Operator129/5
  Alignment33/1 -> Logical Operator155/1, Logical Operator148/4, Logical Operator159/4, Logical Operator157/4, Logical Operator143/4
  Logical Operator130/1 -> Logical Operator129/1
  Logical Operator141/1 -> Logical Operator161/1, Logical Operator149/1, Logical Operator148/1, Logical Operator146/1, Logical Operator152/1, Logical Operator159/1
  Logical Operator119/1 -> Logical Operator139/1, Logical Operator127/1, Logical Operator126/1, Logical Operator124/1, Logical Operator130/1, Logical Operator137/1
  Alignment23/1 -> Logical Operator128/1, Logical Operator135/1, Logical Operator123/1, Logical Operator122/1, Logical Operator121/1, Logical Operator120/1, Logical Operator119/1
  Logical Operator131/1 -> Logical Operator139/2, Logical Operator137/2, Logical Operator130/2, Logical Operator122/2, Logical Operator121/2, Logical Operator120/2
  Alignment29/1 -> Logical Operator156/1, Logical Operator146/5, Logical Operator150/5, Logical Operator152/5, Logical Operator142/5
  Logical Operator156/1 -> Logical Operator161/5, Logical Operator148/5, Logical Operator149/5, Logical Operator159/5, Logical Operator157/5, Logical Operator145/5, Logical Operator144/5, Logical Operator143/5
  Logical Operator138/1 -> Alignment31/1
  Logical Operator123/1 -> Logical Operator138/5
  Alignment36/1 -> Logical Operator83/2, Logical Operator84/2, Logical Operator162/2, Logical Operator158/2, Logical Operator91/2, Logical Operator147/2, Logical Operator87/1
  Logical Operator93/1 -> Alignment27/1
  Alignment35/1 -> Logical Operator90/1, Logical Operator158/5, Logical Operator84/5, Logical Operator86/5, Logical Operator114/5
  Alignment38/1 -> Logical Operator89/1, Logical Operator162/4, Logical Operator92/4, Logical Operator91/4, Logical Operator125/4
  Logical Operator95/1 -> Alignment38/1
  Logical Operator94/1 -> Alignment26/1
  Logical Operator99/1 -> Logical Operator115/4
  Logical Operator121/1 -> Logical Operator138/3
  Alignment21/1 -> Logical Operator105/1, Logical Operator112/1, Logical Operator100/1, Logical Operator99/1, Logical Operator98/1, Logical Operator97/1, Logical Operator96/1
  Logical Operator136/1 -> Logical Operator94/4
  Logical Operator108/1 -> Logical Operator116/2, Logical Operator113/2, Logical Operator107/2, Logical Operator99/2, Logical Operator98/2, Logical Operator97/2
  Logical Operator84/1 -> Logical Operator85/5
  Logical Operator96/1 -> Logical Operator116/1, Logical Operator104/1, Logical Operator102/1, Logical Operator101/1, Logical Operator107/1, Logical Operator113/1
  Logical Operator111/1 -> Logical Operator116/5, Logical Operator102/5, Logical Operator104/5, Logical Operator113/5, Logical Operator112/5, Logical Operator100/5, Logical Operator99/5, Logical Operator98/5
  Logical Operator126/1 -> Logical Operator129/3
  Logical Operator110/1 -> Logical Operator116/4, Logical Operator104/4, Logical Operator105/4, Logical Operator101/4, Logical Operator107/4, Logical Operator100/4, Logical Operator99/4, Logical Operator97/4
  Logical Operator107/1 -> Logical Operator106/1
  Logical Operator102/1 -> Logical Operator106/3
  Logical Operator105/1 -> Logical Operator106/5
  Logical Operator113/1 -> Logical Operator95/2
  Logical Operator100/1 -> Logical Operator115/5
  Logical Operator142/1 -> Logical Operator160/2
  Logical Operator135/1 -> Logical Operator118/1
  Logical Operator127/1 -> Logical Operator129/4
  Logical Operator109/1 -> Logical Operator102/3, Logical Operator105/3, Logical Operator101/3, Logical Operator107/3, Logical Operator113/3, Logical Operator112/3, Logical Operator98/3, Logical Operator97/3
  Logical Operator133/1 -> Logical Operator139/4, Logical Operator127/4, Logical Operator128/4, Logical Operator124/4, Logical Operator130/4, Logical Operator123/4, Logical Operator122/4, Logical Operator120/4
  Logical Operator92/1 -> Logical Operator93/2
  Logical Operator116/1 -> Logical Operator115/1
  Logical Operator90/1 -> Logical Operator117/5, Logical Operator162/5, Logical Operator83/5, Logical Operator92/5, Logical Operator91/5, Logical Operator147/5, Logical Operator136/5, Logical Operator125/5
  Logical Operator85/1 -> Alignment24/1
  Logical Operator104/1 -> Logical Operator106/4
  Logical Operator132/1 -> Logical Operator126/3, Logical Operator128/3, Logical Operator124/3, Logical Operator130/3, Logical Operator137/3, Logical Operator135/3, Logical Operator121/3, Logical Operator120/3
  Logical Operator115/1 -> Alignment37/1
  Logical Operator146/1 -> Logical Operator151/2
  Alignment31/1 -> Logical Operator161/3, Logical Operator145/3, Logical Operator149/3, Logical Operator144/3, Logical Operator154/1
  Logical Operator150/1 -> Logical Operator151/5
  Logical Operator112/1 -> Logical Operator95/1
  Logical Operator139/1 -> Logical Operator138/1
  Alignment30/1 -> Logical Operator149/2, Logical Operator150/2, Logical Operator148/2, Logical Operator146/2, Logical Operator157/2, Logical Operator145/2, Logical Operator153/1
  Logical Operator158/1 -> Logical Operator85/2
  Logical Operator86/1 -> Logical Operator85/1
  Logical Operator147/1 -> Logical Operator94/5
  Logical Operator162/1 -> Logical Operator85/3
  Logical Operator87/1 -> Logical Operator117/2, Logical Operator92/2, Logical Operator86/2, Logical Operator136/2, Logical Operator125/2, Logical Operator114/2
  Logical Operator114/1 -> Logical Operator94/2
  Logical Operator83/1 -> Logical Operator85/4
  Logical Operator91/1 -> Logical Operator93/1
  Alignment37/1 -> Logical Operator117/3, Logical Operator147/3, Logical Operator83/3, Logical Operator136/3, Logical Operator88/1
  Logical Operator159/1 -> Logical Operator140/2
  Logical Operator143/1 -> Logical Operator160/3
  Logical Operator88/1 -> Logical Operator162/3, Logical Operator84/3, Logical Operator158/3, Logical Operator86/3, Logical Operator92/3, Logical Operator91/3, Logical Operator125/3, Logical Operator114/3
  Alignment34/1 -> Logical Operator84/1, Logical Operator91/1, Logical Operator147/1, Logical Operator136/1, Logical Operator125/1, Logical Operator114/1, Logical Operator103/1
  Alignment40/1 -> Logical Operator110/1, Logical Operator102/4, Logical Operator113/4, Logical Operator112/4, Logical Operator98/4
  Alignment22/1 -> Logical Operator111/1, Logical Operator101/5, Logical Operator105/5, Logical Operator107/5, Logical Operator97/5
  Logical Operator89/1 -> Logical Operator117/4, Logical Operator83/4, Logical Operator84/4, Logical Operator158/4, Logical Operator86/4, Logical Operator147/4, Logical Operator136/4, Logical Operator114/4
  Logical Operator120/1 -> Logical Operator138/2
  Alignment32/1 -> Logical Operator104/2, Logical Operator105/2, Logical Operator102/2, Logical Operator101/2, Logical Operator112/2, Logical Operator100/2, Logical Operator108/1
  Logical Operator103/1 -> Logical Operator117/1, Logical Operator83/1, Logical Operator162/1, Logical Operator158/1, Logical Operator86/1, Logical Operator92/1
  Logical Operator153/1 -> Logical Operator161/2, Logical Operator159/2, Logical Operator152/2, Logical Operator144/2, Logical Operator143/2, Logical Operator142/2
  Alignment39/1 -> Logical Operator116/3, Logical Operator100/3, Logical Operator104/3, Logical Operator99/3, Logical Operator109/1
  Logical Operator101/1 -> Logical Operator106/2
  Logical Operator134/1 -> Logical Operator139/5, Logical Operator126/5, Logical Operator127/5, Logical Operator137/5, Logical Operator135/5, Logical Operator123/5, Logical Operator122/5, Logical Operator121/5
  Logical Operator98/1 -> Logical Operator115/3
  Logical Operator97/1 -> Logical Operator115/2
  Logical Operator122/1 -> Logical Operator138/4
  Logical Operator125/1 -> Logical Operator94/3
  Logical Operator81/1 -> Alignment39/1
  Logical Operator63/1 -> Alignment40/1
  Logical Operator73/1 -> Alignment22/1
  Bus Selector1/8 -> Alignment2/1  "<b0>"
  Bus Selector2/8 -> Alignment1/1  "<b0>"
  Bus Selector2/6 -> Alignment11/1  "<b2>"
  Bus Selector2/5 -> Alignment16/1  "<b3>"
  Bus Selector2/4 -> Alignment21/1  "<b4>"
  Bus Selector2/3 -> Alignment34/1  "<b5>"
  Bus Selector2/2 -> Alignment23/1  "<b6>"
  Bus Selector2/1 -> Alignment28/1, "A is negative B is positive "/2, Logical Operator303/1, Logical Operator327/1  "<b7>"
  Bus Selector1/6 -> Alignment13/1  "<b2>"
  Bus Selector1/5 -> Alignment18/1  "<b3>"
  Bus Selector1/4 -> Alignment32/1  "<b4>"
  Bus Selector1/3 -> Alignment36/1  "<b5>"
  Bus Selector1/2 -> Alignment25/1  "<b6>"
  Bus Selector1/1 -> Alignment30/1, A is positive B is negative/2, Logical Operator325/1, Logical Operator/2  "<b7>"
  Logical Operator140/1 -> A = B(1b)/1
  Logical Operator151/1 -> (uint) A < B(1b)/1, Enable unsigned (A < B)/2
  Logical Operator160/1 -> Enable unsigned (2) (A > B)/1, (uint) A > B(1b)/1
  Logical Operator/1 -> Logical Operator326/1
  Logical Operator327/1 -> Logical Operator/1
  Logical Operator325/1 -> Logical Operator303/2
  Logical Operator303/1 -> Logical Operator326/2
  A(1B)/1 -> Bus Selector2/1
  B(1B)/1 -> Bus Selector1/1

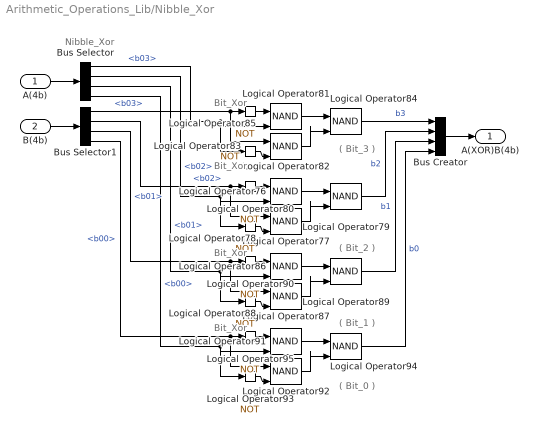
== system Arithmetic_Operations_Lib/Nibble_Xor ==
  note: Nibble_Xor
  note: Bit_Xor
  note: ( Bit_0 )
  note: ( Bit_1 )
  note: Bit_Xor
  note: ( Bit_2 )
  note: ( Bit_3 )
  note: Bit_Xor
  note: Bit_Xor
  A(4b) : Inport
  B(4b) : Inport  Port=2
  Bus Creator : BusCreator  Inputs=4
  Bus Selector : BusSelector  OutputSignals=b03,b02,b01,b00
  Bus Selector1 : BusSelector  OutputSignals=b03,b02,b01,b00
  Logical Operator{76..77,79,81..82,84,86..87,89,91..92,94} (12 alike) : Logic  Operator=NAND  IconShape=distinctive  AllPortsSameDT=off  OutDataTypeStr=boolean
  Logical Operator{78,80,83,85,88,90,93,95} (8 alike) : Logic  Operator=NOT  IconShape=distinctive  AllPortsSameDT=off  OutDataTypeStr=boolean
  A(XOR)B(4b) : Outport  OutputWhenDisabled=reset
  wires:
  Logical Operator83/1 -> Logical Operator82/2
  Logical Operator78/1 -> Logical Operator77/2
  Logical Operator90/1 -> Logical Operator86/1
  Logical Operator88/1 -> Logical Operator87/2
  Logical Operator79/1 -> Bus Creator/2  "b2"
  Logical Operator89/1 -> Bus Creator/3  "b1"
  Bus Selector1/3 -> Logical Operator87/1, Logical Operator90/1  "<b01>"
  Logical Operator86/1 -> Logical Operator89/1
  Bus Selector/1 -> Logical Operator83/1, Logical Operator81/2  "<b03>"
  Bus Selector/3 -> Logical Operator88/1, Logical Operator86/2  "<b01>"
  Logical Operator87/1 -> Logical Operator89/2
  Logical Operator81/1 -> Logical Operator84/1
  Bus Selector1/1 -> Logical Operator85/1, Logical Operator82/1  "<b03>"
  Bus Selector/4 -> Logical Operator93/1, Logical Operator91/2  "<b00>"
  Logical Operator92/1 -> Logical Operator94/2
  Logical Operator76/1 -> Logical Operator79/1
  Logical Operator84/1 -> Bus Creator/1  "b3"
  Logical Operator85/1 -> Logical Operator81/1
  Logical Operator82/1 -> Logical Operator84/2
  Logical Operator95/1 -> Logical Operator91/1
  Logical Operator93/1 -> Logical Operator92/2
  Logical Operator77/1 -> Logical Operator79/2
  Bus Selector1/2 -> Logical Operator77/1, Logical Operator80/1  "<b02>"
  Logical Operator94/1 -> Bus Creator/4  "b0"
  Logical Operator80/1 -> Logical Operator76/1
  Logical Operator91/1 -> Logical Operator94/1
  Bus Selector/2 -> Logical Operator78/1, Logical Operator76/2  "<b02>"
  Bus Selector1/4 -> Logical Operator95/1, Logical Operator92/1  "<b00>"
  Bus Creator/1 -> A(XOR)B(4b)/1
  B(4b)/1 -> Bus Selector1/1
  A(4b)/1 -> Bus Selector/1
